simulink model "uncontrolled"  (R2021a)
settings: Solver=ode15s  StartTime=0  StopTime=6043.3926  MaxStep=0.0038168  RelTol=1e-8  AbsTol=1e-8
values from neighbouring files (symbols this model uses):
  I_x = 91.6*1e-2    (= 0.916)    [DATA.m]
  I_y = 25.1*1e-2    (= 0.251)    [DATA.m]
  I_z = 100.9*1e-2    (= 1.009)    [DATA.m]
  mag_ind = [0.1 0.5 0.1]'    [DATA.m]
  mu_E = 398600    [DATA.m]
  n_sun = 2*pi/365/24/3600    (= 1.99238499086e-07)    [DATA.m]
  phi0_312 = -atan(A_313_0(2,1)/A_313_0(2,2))    [DATA.m]
  phi0_313 = deg2rad(9.7)    [DATA.m]
  psi0_312 = -atan(A_313_0(1,3)/A_313_0(3,3))    [DATA.m]
  psi0_313 = deg2rad(6)    [DATA.m]
  R_E = 6.3710e3    (= 6371)    [DATA.m]
  th0_312 = asin(A_313_0(2,3))    [DATA.m]
  th0_313 = deg2rad(19)    [DATA.m]
  w_E = 2*pi/24/3600    (= 7.27220521664e-05)    [DATA.m]
undefined symbols (not defined in the file or in its folder): orbit, SRP
libraries: lib x11, vrlib x1, simulink_extras x1
settings Model: Creator=dvd33  LastModifiedBy=dvd33
settings SolverCC: AlgebraicLoopSolver=TrustRegion  ODENIntegrationMethod=ode4
settings DebuggingCC: IgnoredZcDiagnostic=none  SFMachineParentedDataDiag=warning

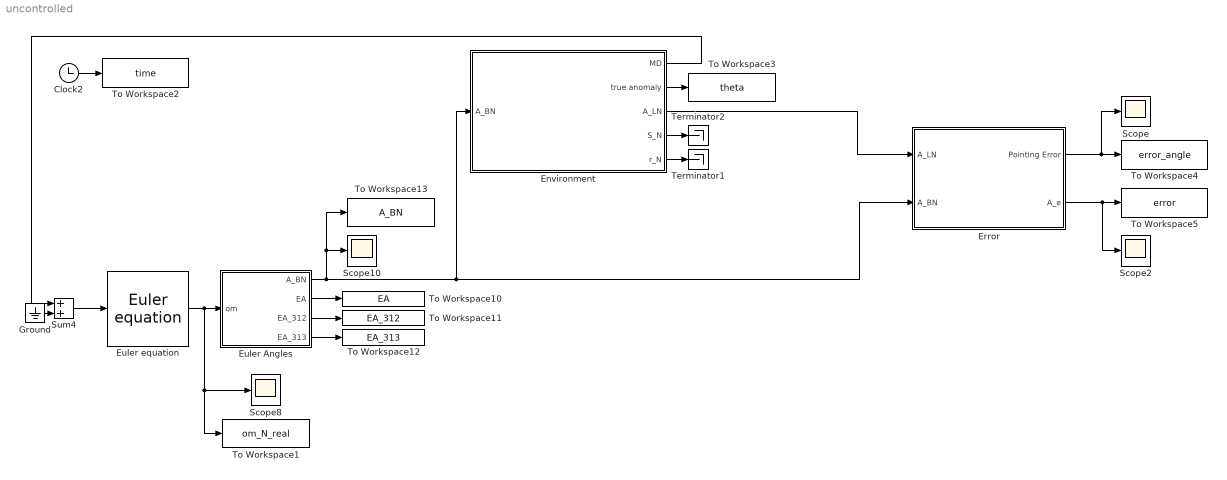
== system uncontrolled ==
  Clock2 : Clock
  Environment : Subsystem
  Error : Subsystem
  Euler Angles : Subsystem
  Euler equation : lib/Euler equation  SystemSampleTime=-1  VariantActivationTime=update diagram  Latency=0  AutoFrameSizeCalculation=off
  Ground : Ground
  Scope{,2,8,10} (4 alike) : Scope
  Sum4 : Sum
  Terminator1 : Terminator
  Terminator2 : Terminator
  To Workspace1 : ToWorkspace  VariableName=om_N_real  SampleTime=-1
  To Workspace10 : ToWorkspace  VariableName=EA  SampleTime=-1
  To Workspace11 : ToWorkspace  VariableName=EA_312  SampleTime=-1
  To Workspace12 : ToWorkspace  VariableName=EA_313  SampleTime=-1
  To Workspace13 : ToWorkspace  VariableName=A_BN  SampleTime=-1
  To Workspace2 : ToWorkspace  VariableName=time  SampleTime=-1
  To Workspace3 : ToWorkspace  VariableName=theta  SampleTime=-1
  To Workspace4 : ToWorkspace  VariableName=error_angle  SampleTime=-1
  To Workspace5 : ToWorkspace  VariableName=error  SampleTime=-1
  wires:
  Euler Angles/3(EA_312) -> To Workspace11/1
  Euler Angles/4(EA_313) -> To Workspace12/1
  Euler Angles/2(EA) -> To Workspace10/1
  Euler equation/1 -> Euler Angles/1(om), To Workspace1/1, Scope8/1
  Environment/2(true anomaly) -> To Workspace3/1
  Environment/3(A_LN) -> Error/1(A_LN)
  Environment/1(MD) -> Sum4/1
  Error/2(A_e) -> Scope2/1, To Workspace5/1
  Euler Angles/1(A_BN) -> Environment/1(A_BN), Error/2(A_BN), To Workspace13/1, Scope10/1
  Error/1(Pointing Error) -> To Workspace4/1, Scope/1
  Clock2/1 -> To Workspace2/1
  Sum4/1 -> Euler equation/1
  Ground/1 -> Sum4/2
  Environment/4(S_N) -> Terminator2/1
  Environment/5(r_N) -> Terminator1/1

== system uncontrolled/Environment ==
  A_BN : Inport
  A_BN1 : InportShadow
  Disturbance torques : Subsystem
  Orbit and Sun : Subsystem
  MD : Outport
  true anomaly : Outport  Port=2
  A_LN : Outport  Port=3
  S_N : Outport  Port=4
  r_N : Outport  Port=5
  wires:
  Orbit and Sun/1(r_N) -> r_N/1, Disturbance torques/1(r_N)
  Orbit and Sun/3(true anomaly) -> true anomaly/1
  A_BN/1 -> Orbit and Sun/1(A_BN)
  Disturbance torques/1(MD) -> MD/1
  Orbit and Sun/2(A_LN) -> A_LN/1, Disturbance torques/2(A_LN)
  Orbit and Sun/4(S_B) -> Disturbance torques/4(S_B)
  Orbit and Sun/5(S_N) -> S_N/1
  A_BN1/1 -> Disturbance torques/3(A_BN)

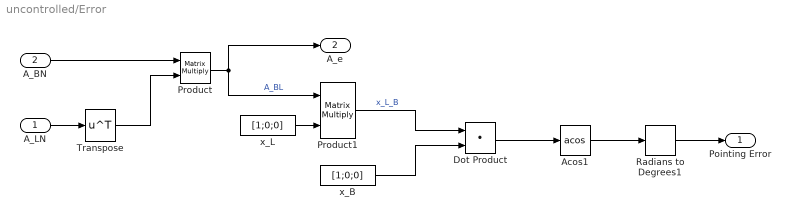
== system uncontrolled/Error ==
  A_LN : Inport
  A_BN : Inport  Port=2
  Acos1 : Trigonometry  Operator=acos
  Dot Product : DotProduct  InputSameDT=on  OutDataTypeStr=Inherit: Inherit via internal rule
  Product : Product  Multiplication=Matrix(*)
  Product1 : Product  Multiplication=Matrix(*)
  Radians to Degrees1 : simulink_extras/Transformations/Radians to Degrees
  Transpose : Math  Operator=transpose  SaturateOnIntegerOverflow=on
  x_B : Constant  Value=[1;0;0]
  x_L : Constant  Value=[1;0;0]
  Pointing Error : Outport
  A_e : Outport  Port=2
  wires:
  A_LN/1 -> Transpose/1
  A_BN/1 -> Product/1
  Transpose/1 -> Product/2
  Product/1 -> Product1/1, A_e/1  "A_BL"
  Radians to Degrees1/1 -> Pointing Error/1
  x_L/1 -> Product1/2
  Dot Product/1 -> Acos1/1
  Acos1/1 -> Radians to Degrees1/1
  Product1/1 -> Dot Product/1  "x_L_B"
  x_B/1 -> Dot Product/2

== system uncontrolled/Euler Angles ==
  om : Inport
  312 : Subsystem  TreatAsAtomicUnit=on
  313 : Subsystem  TreatAsAtomicUnit=on
  Abs : Abs
  SWITCH : Subsystem
  Selector2 : Selector  NumberOfDimensions=2  InputPortWidth=3,3  IndexOptions=Index vector (dialog),Index vector (dialog)  Indices=3,3  OutputSizes=1,1
  A_BN : Outport
  EA : Outport  Port=2
  EA_312 : Outport  Port=3
  EA_313 : Outport  Port=4
  wires:
  om/1 -> 313/1(om), 312/1(om)
  Selector2/1 -> Abs/1  "cos(th)"
  312/2(EA) -> SWITCH/2(EA_312), EA_312/1
  313/2(EA) -> SWITCH/5(EA_313), EA_313/1
  313/1(A_BN_313) -> Selector2/1, SWITCH/4(A_BN_313)
  312/1(A_BN_312) -> SWITCH/1(A_BN_312)
  Abs/1 -> SWITCH/3(u1)
  SWITCH/1(EA) -> EA/1
  SWITCH/2(A_BN) -> A_BN/1

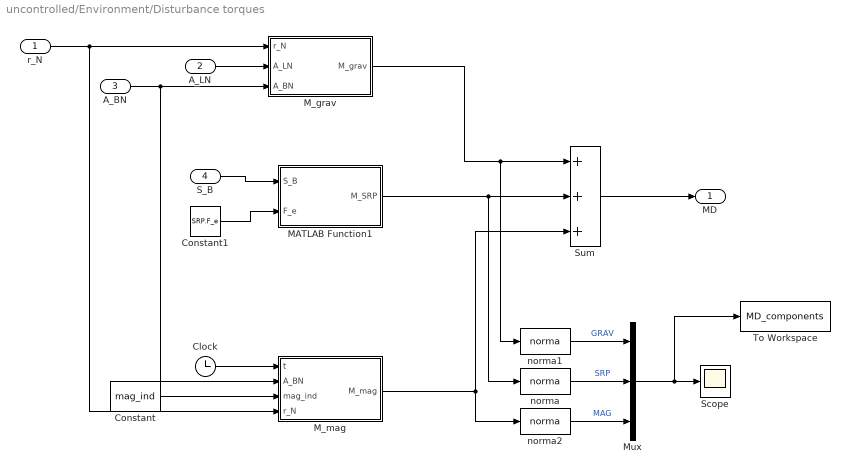
== system uncontrolled/Environment/Disturbance torques ==
  r_N : Inport
  A_LN : Inport  Port=2
  A_BN : Inport  Port=3
  S_B : Inport  Port=4
  Clock : Clock
  Constant : Constant  Value=mag_ind
  Constant1 : Constant  Value=SRP.F_e
  MATLAB Function1 : MATLAB Function  TreatAsAtomicUnit=on
  M_grav : Subsystem
  M_mag : Subsystem
  Mux : Mux  Inputs=3
  Scope : Scope
  Sum : Sum  Inputs=+++
  To Workspace : ToWorkspace  VariableName=MD_components  SampleTime=-1
  norma : lib/norma  SystemSampleTime=-1  VariantActivationTime=update diagram  Latency=0  AutoFrameSizeCalculation=off
  norma1 : lib/norma  SystemSampleTime=-1  VariantActivationTime=update diagram  Latency=0  AutoFrameSizeCalculation=off
  norma2 : lib/norma  SystemSampleTime=-1  VariantActivationTime=update diagram  Latency=0  AutoFrameSizeCalculation=off
  MD : Outport
  wires:
  r_N/1 -> M_grav/1(r_N), M_mag/4(r_N)
  A_LN/1 -> M_grav/2(A_LN)
  A_BN/1 -> M_mag/2(A_BN), M_grav/3(A_BN)
  Sum/1 -> MD/1
  M_grav/1(M_grav) -> norma1/1, Sum/1
  S_B/1 -> MATLAB Function1/1(S_B)
  MATLAB Function1/1(M_SRP) -> Sum/2, norma/1
  M_mag/1(M_mag) -> norma2/1, Sum/3
  Clock/1 -> M_mag/1(t)
  Constant/1 -> M_mag/3(mag_ind)
  Mux/1 -> To Workspace/1, Scope/1
  norma1/1 -> Mux/1  "GRAV"
  norma2/1 -> Mux/3  "MAG"
  norma/1 -> Mux/2  "SRP"
  Constant1/1 -> MATLAB Function1/2(F_e)

== system uncontrolled/Environment/Orbit and Sun ==
  A_BN : Inport
  Clock : Clock
  Orbit : Subsystem
  Product : Product  Multiplication=Matrix(*)
  Subsystem : Subsystem
  Sun direction : Subsystem
  r_N : Outport
  A_LN : Outport  Port=2
  true anomaly : Outport  Port=3
  S_B : Outport  Port=4
  S_N : Outport  Port=5
  wires:
  A_BN/1 -> Product/1
  Orbit/2(true anomaly) -> Subsystem/1(theta), true anomaly/1
  Orbit/1(r_N) -> r_N/1
  Clock/1 -> Sun direction/1(t)
  Sun direction/1(S_N) -> Product/2, S_N/1
  Product/1 -> S_B/1
  Subsystem/1(A_LN) -> A_LN/1

== system uncontrolled/Euler Angles/312 ==
  om : Inport
  A_312 : Subsystem
  Angles 312 : Subsystem
  A_BN_312 : Outport
  EA : Outport  Port=2
  wires:
  Angles 312/1(EA) -> A_312/1(EA), EA/1
  om/1 -> Angles 312/1(om)
  A_312/1(A_BN_312) -> A_BN_312/1

== system uncontrolled/Euler Angles/313 ==
  om : Inport
  A_313 : Subsystem
  Angles 313 : Subsystem
  A_BN_313 : Outport
  EA : Outport  Port=2
  wires:
  Angles 313/1(EA) -> A_313/1(EA), EA/1
  A_313/1(A_BN_313) -> A_BN_313/1
  om/1 -> Angles 313/1(om)

== system uncontrolled/Euler Angles/SWITCH ==
  A_BN_312 : Inport
  EA_312 : Inport  Port=2
  u1 : Inport  Port=3
  A_BN_313 : Inport  Port=4
  EA_313 : Inport  Port=5
  Switch : Switch  Criteria=u2 > Threshold  Threshold=0.9999
  Switch2 : Switch  Criteria=u2 > Threshold  Threshold=0.9999
  u1_1 : InportShadow  Port=3
  EA : Outport
  A_BN : Outport  Port=2
  wires:
  u1/1 -> Switch2/2
  Switch2/1 -> A_BN/1
  Switch/1 -> EA/1
  EA_312/1 -> Switch/1
  EA_313/1 -> Switch/3
  A_BN_312/1 -> Switch2/1
  A_BN_313/1 -> Switch2/3
  u1_1/1 -> Switch/2

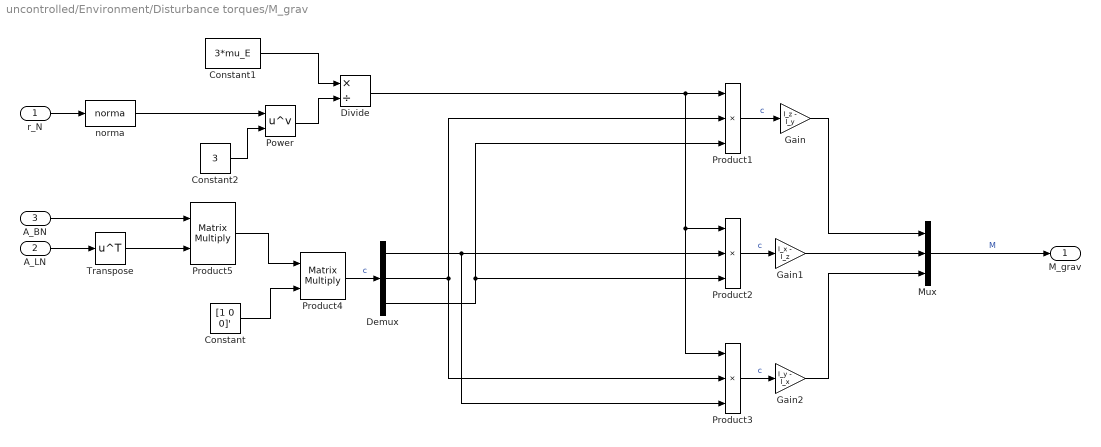
== system uncontrolled/Environment/Disturbance torques/M_grav ==
  r_N : Inport
  A_LN : Inport  Port=2
  A_BN : Inport  Port=3
  Constant : Constant  Value=[1 0 0]'
  Constant1 : Constant  Value=3*mu_E
  Constant2 : Constant  Value=3
  Demux : Demux  Outputs=3
  Divide : Product  Inputs=*/
  Gain : Gain  Gain=I_z - I_y
  Gain1 : Gain  Gain=I_x - I_z
  Gain2 : Gain  Gain=I_y - I_x
  Mux : Mux  Inputs=3
  Power : Math  Operator=pow  SaturateOnIntegerOverflow=on
  Product1 : Product  Inputs=3
  Product2 : Product  Inputs=3
  Product3 : Product  Inputs=3
  Product4 : Product  Multiplication=Matrix(*)
  Product5 : Product  Multiplication=Matrix(*)
  Transpose : Math  Operator=transpose  SaturateOnIntegerOverflow=on
  norma : lib/norma  SystemSampleTime=-1  VariantActivationTime=update diagram  Latency=0  AutoFrameSizeCalculation=off
  M_grav : Outport
  wires:
  A_LN/1 -> Transpose/1
  Demux/1 -> Product2/2, Product3/3
  Product2/1 -> Gain1/1  "c"
  Constant/1 -> Product4/2
  Product5/1 -> Product4/1
  Transpose/1 -> Product5/2
  Mux/1 -> M_grav/1  "M"
  Product1/1 -> Gain/1  "c"
  Constant1/1 -> Divide/1
  Product3/1 -> Gain2/1  "c"
  Power/1 -> Divide/2
  Demux/2 -> Product3/2, Product1/2
  Divide/1 -> Product1/1, Product2/1, Product3/1
  Constant2/1 -> Power/2
  Demux/3 -> Product1/3, Product2/3
  Product4/1 -> Demux/1  "c"
  A_BN/1 -> Product5/1
  r_N/1 -> norma/1
  norma/1 -> Power/1
  Gain/1 -> Mux/1
  Gain1/1 -> Mux/2
  Gain2/1 -> Mux/3

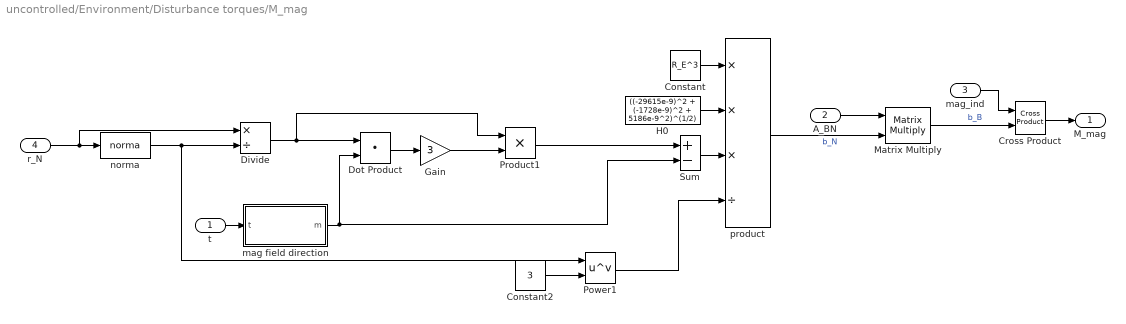
== system uncontrolled/Environment/Disturbance torques/M_mag ==
  t : Inport
  A_BN : Inport  Port=2
  mag_ind : Inport  Port=3
  r_N : Inport  Port=4
  Constant : Constant  Value=R_E^3
  Constant2 : Constant  Value=3
  Cross Product : vrlib/Utilities/Cross Product
  Divide : Product  Inputs=*/
  Dot Product : DotProduct  InputSameDT=on  OutDataTypeStr=Inherit: Inherit via internal rule
  Gain : Gain  Gain=3
  H0 : Constant  Value=((-29615e-9)^2 + (-1728e-9)^2 + 5186e-9^2)^(1/2)
  Matrix Multiply : Product  Multiplication=Matrix(*)
  Power1 : Math  Operator=pow  SaturateOnIntegerOverflow=on
  Product1 : Product
  Sum : Sum  Inputs=+-
  mag field direction : Subsystem
  norma : lib/norma  SystemSampleTime=-1  VariantActivationTime=update diagram  Latency=0  AutoFrameSizeCalculation=off
  product : Product  Inputs=***/
  M_mag : Outport
  wires:
  t/1 -> mag field direction/1(t)
  A_BN/1 -> Matrix Multiply/1
  Constant/1 -> product/1
  Power1/1 -> product/4
  Constant2/1 -> Power1/2
  norma/1 -> Power1/1, Divide/2
  Divide/1 -> Product1/1, Dot Product/1
  H0/1 -> product/2
  Dot Product/1 -> Gain/1
  Gain/1 -> Product1/2
  Sum/1 -> product/3
  product/1 -> Matrix Multiply/2  "b_N"
  r_N/1 -> Divide/1, norma/1
  mag field direction/1(m) -> Dot Product/2, Sum/2
  Cross Product/1 -> M_mag/1
  Product1/1 -> Sum/1
  Matrix Multiply/1 -> Cross Product/2  "b_B"
  mag_ind/1 -> Cross Product/1

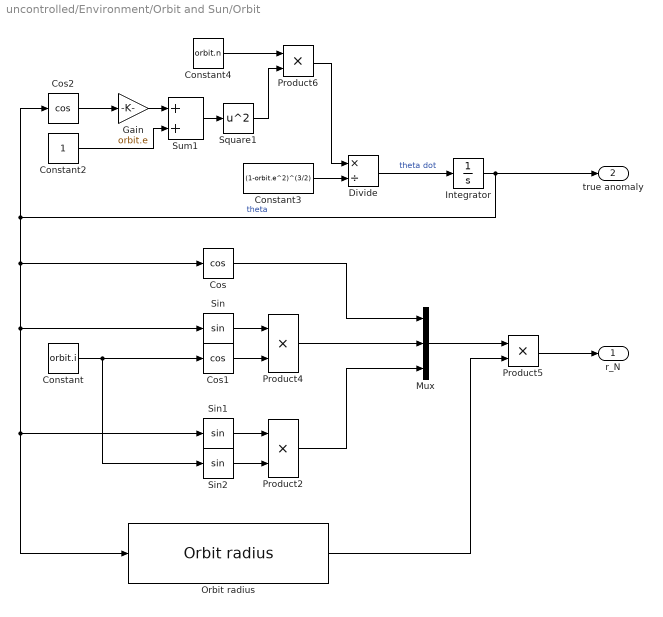
== system uncontrolled/Environment/Orbit and Sun/Orbit ==
  Constant : Constant  Value=orbit.i
  Constant2 : Constant
  Constant3 : Constant  Value=(1-orbit.e^2)^(3/2)
  Constant4 : Constant  Value=orbit.n
  Cos : Trigonometry  Operator=cos
  Cos1 : Trigonometry  Operator=cos
  Cos2 : Trigonometry  Operator=cos
  Divide : Product  Inputs=*/
  Gain : Gain  Gain=orbit.e
  Integrator : Integrator  InitialCondition=orbit.theta0
  Mux : Mux  Inputs=3
  Orbit radius : lib/Orbit radius  SystemSampleTime=-1  VariantActivationTime=update diagram  Latency=0  AutoFrameSizeCalculation=off
      link override Constant: Value=orbit.a*(1-orbit.e^2)
      link override eccentricity: Value=orbit.e
  Product{2,4..6} (4 alike) : Product
  Sin : Trigonometry
  Sin1 : Trigonometry
  Sin2 : Trigonometry
  Square1 : Math  Operator=square  SaturateOnIntegerOverflow=on
  Sum1 : Sum
  r_N : Outport
  true anomaly : Outport  Port=2
  wires:
  Divide/1 -> Integrator/1  "theta dot"
  Integrator/1 -> true anomaly/1, Cos2/1, Sin/1, Orbit radius/1, Sin1/1, Cos/1  "theta"
  Product2/1 -> Mux/3
  Constant2/1 -> Sum1/2
  Product5/1 -> r_N/1
  Sin1/1 -> Product2/1
  Orbit radius/1 -> Product5/2
  Constant4/1 -> Product6/1
  Square1/1 -> Product6/2
  Sum1/1 -> Square1/1
  Gain/1 -> Sum1/1
  Cos1/1 -> Product4/2
  Product4/1 -> Mux/2
  Cos2/1 -> Gain/1
  Product6/1 -> Divide/1
  Constant3/1 -> Divide/2
  Constant/1 -> Sin2/1, Cos1/1
  Sin2/1 -> Product2/2
  Cos/1 -> Mux/1
  Mux/1 -> Product5/1
  Sin/1 -> Product4/1

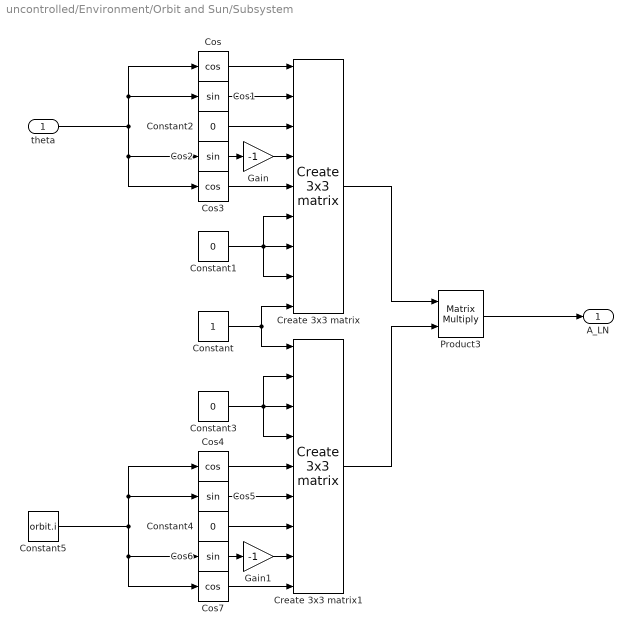
== system uncontrolled/Environment/Orbit and Sun/Subsystem ==
  theta : Inport
  Constant : Constant
  Constant{1..4} (4 alike) : Constant  Value=0
  Constant5 : Constant  Value=orbit.i
  Cos{,3..4,7} (4 alike) : Trigonometry  Operator=cos
  Cos{1..2,5..6} (4 alike) : Trigonometry
  Create 3x3 matrix : lib/Create 3x3 matrix  SystemSampleTime=-1  VariantActivationTime=update diagram  Latency=0  AutoFrameSizeCalculation=off
  Create 3x3 matrix1 : lib/Create 3x3 matrix  SystemSampleTime=-1  VariantActivationTime=update diagram  Latency=0  AutoFrameSizeCalculation=off
  Gain : Gain  Gain=-1
  Gain1 : Gain  Gain=-1
  Product3 : Product  Multiplication=Matrix(*)
  A_LN : Outport
  wires:
  Create 3x3 matrix1/1 -> Product3/2
  Create 3x3 matrix/1 -> Product3/1
  Product3/1 -> A_LN/1
  Cos/1 -> Create 3x3 matrix/1
  Cos1/1 -> Create 3x3 matrix/2
  Cos3/1 -> Create 3x3 matrix/5
  Cos2/1 -> Gain/1
  Gain/1 -> Create 3x3 matrix/4
  Constant/1 -> Create 3x3 matrix1/1, Create 3x3 matrix/9
  Constant1/1 -> Create 3x3 matrix/6, Create 3x3 matrix/7, Create 3x3 matrix/8
  Constant2/1 -> Create 3x3 matrix/3
  Constant3/1 -> Create 3x3 matrix1/2, Create 3x3 matrix1/3, Create 3x3 matrix1/4
  Cos5/1 -> Create 3x3 matrix1/6
  Cos4/1 -> Create 3x3 matrix1/5
  Constant4/1 -> Create 3x3 matrix1/7
  Cos7/1 -> Create 3x3 matrix1/9
  Cos6/1 -> Gain1/1
  Gain1/1 -> Create 3x3 matrix1/8
  theta/1 -> Cos2/1, Cos3/1, Cos/1, Cos1/1
  Constant5/1 -> Cos6/1, Cos7/1, Cos5/1, Cos4/1

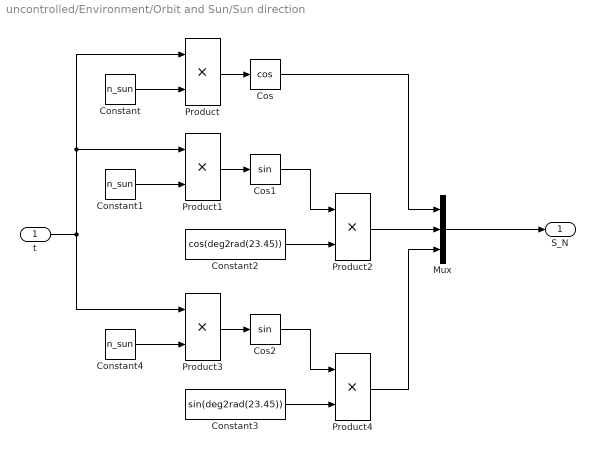
== system uncontrolled/Environment/Orbit and Sun/Sun direction ==
  t : Inport
  Constant : Constant  Value=n_sun
  Constant1 : Constant  Value=n_sun
  Constant2 : Constant  Value=cos(deg2rad(23.45))
  Constant3 : Constant  Value=sin(deg2rad(23.45))
  Constant4 : Constant  Value=n_sun
  Cos : Trigonometry  Operator=cos
  Cos1 : Trigonometry
  Cos2 : Trigonometry
  Mux : Mux  Inputs=3
  Product{,1..4} (5 alike) : Product
  S_N : Outport
  wires:
  Mux/1 -> S_N/1
  Constant/1 -> Product/2
  Product/1 -> Cos/1
  Cos/1 -> Mux/1
  Product1/1 -> Cos1/1
  Constant1/1 -> Product1/2
  Cos1/1 -> Product2/1
  Constant2/1 -> Product2/2
  Product2/1 -> Mux/2
  t/1 -> Product3/1, Product1/1, Product/1
  Product4/1 -> Mux/3
  Cos2/1 -> Product4/1
  Constant4/1 -> Product3/2
  Product3/1 -> Cos2/1
  Constant3/1 -> Product4/2

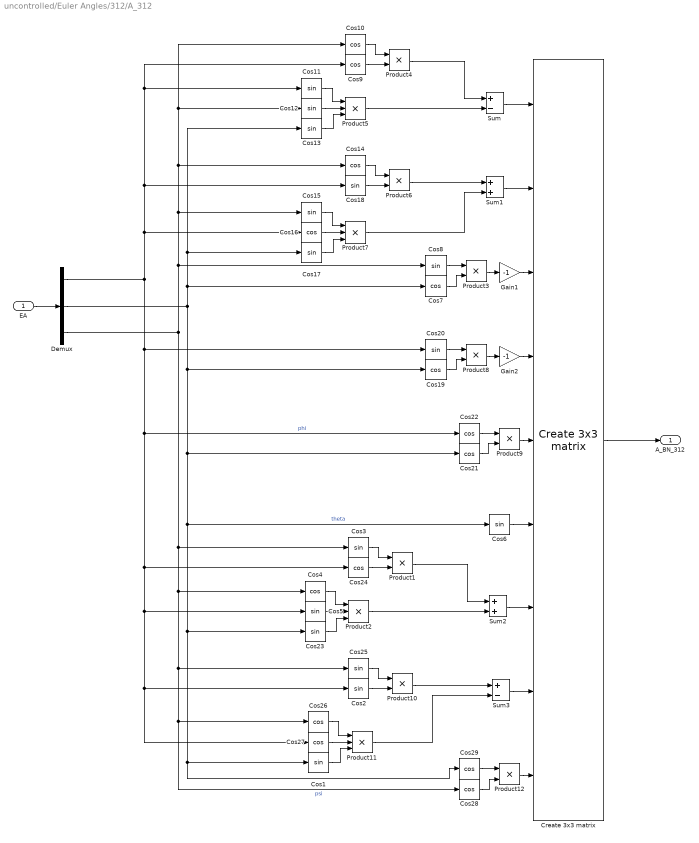
== system uncontrolled/Euler Angles/312/A_312 ==
  EA : Inport
  Cos{1..3,5..6,8,11..13,15,17..18,20,23,25} (15 alike) : Trigonometry
  Cos{4,7,9..10,14,16,19,21..22,24,26..29} (14 alike) : Trigonometry  Operator=cos
  Create 3x3 matrix : lib/Create 3x3 matrix  SystemSampleTime=-1  VariantActivationTime=update diagram  Latency=0  AutoFrameSizeCalculation=off
  Demux : Demux  Outputs=3
  Gain1 : Gain  Gain=-1
  Gain2 : Gain  Gain=-1
  Product{1,3..4,6,8..10,12} (8 alike) : Product
  Product{2,5,7,11} (4 alike) : Product  Inputs=3
  Sum : Sum  Inputs=+-
  Sum1 : Sum
  Sum2 : Sum
  Sum3 : Sum  Inputs=+-
  A_BN_312 : Outport
  wires:
  EA/1 -> Demux/1
  Demux/1 -> Cos24/1, Cos5/1, Cos27/1, Cos2/1, Cos22/1, Cos20/1, Cos16/1, Cos18/1, Cos9/1, Cos11/1  "phi"
  Demux/3 -> Cos8/1, Cos15/1, Cos14/1, Cos10/1, Cos12/1, Cos3/1, Cos4/1, Cos25/1, Cos26/1, Cos28/1  "psi"
  Demux/2 -> Cos1/1, Cos29/1, Cos23/1, Cos6/1, Cos21/1, Cos19/1, Cos7/1, Cos13/1, Cos17/1  "theta"
  Product12/1 -> Create 3x3 matrix/9
  Cos29/1 -> Product12/1
  Cos28/1 -> Product12/2
  Sum3/1 -> Create 3x3 matrix/8
  Cos27/1 -> Product11/2
  Product11/1 -> Sum3/2
  Cos25/1 -> Product10/1
  Product10/1 -> Sum3/1
  Cos2/1 -> Product10/2
  Cos26/1 -> Product11/1
  Cos1/1 -> Product11/3
  Cos23/1 -> Product2/3
  Cos4/1 -> Product2/1
  Product2/1 -> Sum2/2
  Cos5/1 -> Product2/2
  Cos24/1 -> Product1/2
  Product1/1 -> Sum2/1
  Cos3/1 -> Product1/1
  Sum2/1 -> Create 3x3 matrix/7
  Product9/1 -> Create 3x3 matrix/5
  Cos22/1 -> Product9/1
  Cos21/1 -> Product9/2
  Product8/1 -> Gain2/1
  Cos20/1 -> Product8/1
  Cos19/1 -> Product8/2
  Gain1/1 -> Create 3x3 matrix/3
  Create 3x3 matrix/1 -> A_BN_312/1
  Product6/1 -> Sum1/1
  Sum/1 -> Create 3x3 matrix/1
  Cos7/1 -> Product3/2
  Cos8/1 -> Product3/1
  Gain2/1 -> Create 3x3 matrix/4
  Cos9/1 -> Product4/2
  Sum1/1 -> Create 3x3 matrix/2
  Product4/1 -> Sum/1
  Cos12/1 -> Product5/2
  Product5/1 -> Sum/2
  Cos11/1 -> Product5/1
  Cos17/1 -> Product7/3
  Cos14/1 -> Product6/1
  Cos6/1 -> Create 3x3 matrix/6
  Cos13/1 -> Product5/3
  Product7/1 -> Sum1/2
  Product3/1 -> Gain1/1
  Cos16/1 -> Product7/2
  Cos15/1 -> Product7/1
  Cos18/1 -> Product6/2
  Cos10/1 -> Product4/1

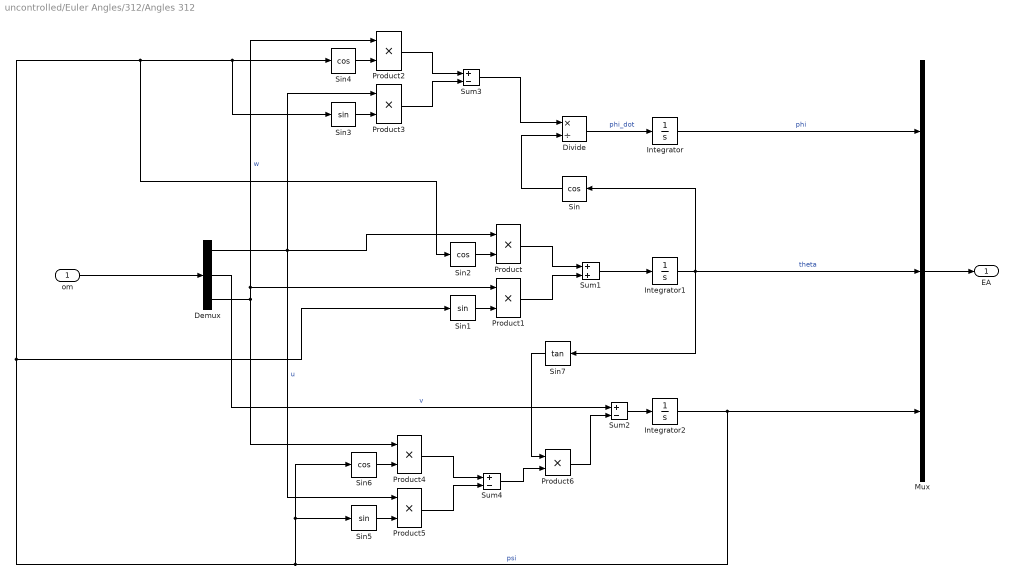
== system uncontrolled/Euler Angles/312/Angles 312 ==
  om : Inport
  Demux : Demux  Outputs=3
  Divide : Product  Inputs=*/
  Integrator : Integrator  InitialCondition=phi0_312  WrapState=on
  Integrator1 : Integrator  InitialCondition=th0_312  WrapState=on
  Integrator2 : Integrator  InitialCondition=psi0_312  WrapState=on
  Mux : Mux  Inputs=3
  Product{,1..6} (7 alike) : Product
  Sin{,2,4,6} (4 alike) : Trigonometry  Operator=cos
  Sin1 : Trigonometry
  Sin3 : Trigonometry
  Sin5 : Trigonometry
  Sin7 : Trigonometry  Operator=tan
  Sum1 : Sum
  Sum2 : Sum  Inputs=+-
  Sum3 : Sum  Inputs=+-
  Sum4 : Sum  Inputs=+-
  EA : Outport
  wires:
  Mux/1 -> EA/1
  Sum4/1 -> Product6/2
  Demux/2 -> Sum2/1  "v"
  Integrator2/1 -> Mux/3, Sin6/1, Sin5/1, Sin3/1, Sin4/1, Sin2/1, Sin1/1  "psi"
  Demux/3 -> Product2/1, Product1/1, Product4/1  "w"
  Sin4/1 -> Product2/2
  Product1/1 -> Sum1/2
  Sin1/1 -> Product1/2
  Sin3/1 -> Product3/2
  Divide/1 -> Integrator/1  "phi_dot"
  Sum1/1 -> Integrator1/1
  Product6/1 -> Sum2/2
  Sin5/1 -> Product5/2
  om/1 -> Demux/1
  Product4/1 -> Sum4/1
  Sum3/1 -> Divide/1
  Product5/1 -> Sum4/2
  Sin6/1 -> Product4/2
  Integrator1/1 -> Sin/1, Mux/2, Sin7/1  "theta"
  Integrator/1 -> Mux/1  "phi"
  Product3/1 -> Sum3/2
  Demux/1 -> Product3/1, Product/1, Product5/1  "u"
  Sin/1 -> Divide/2
  Product/1 -> Sum1/1
  Sin7/1 -> Product6/1
  Product2/1 -> Sum3/1
  Sum2/1 -> Integrator2/1
  Sin2/1 -> Product/2

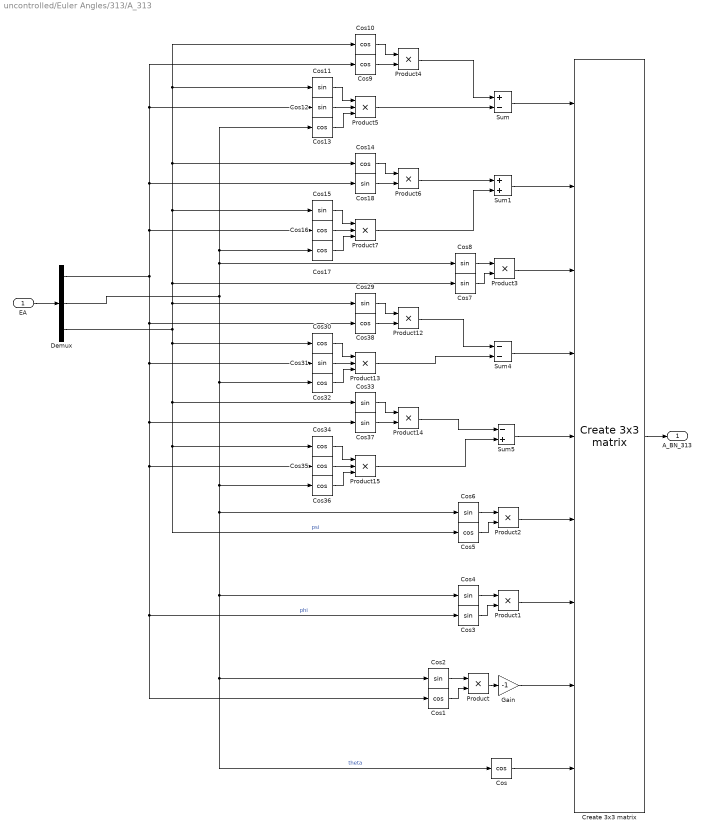
== system uncontrolled/Euler Angles/313/A_313 ==
  EA : Inport
  Cos{,1,5,9..10,13..14,16..17,30,32,34..36,38} (15 alike) : Trigonometry  Operator=cos
  Cos{2..4,6..8,11..12,15,18,29,31,33,37} (14 alike) : Trigonometry
  Create 3x3 matrix : lib/Create 3x3 matrix  SystemSampleTime=-1  VariantActivationTime=update diagram  Latency=0  AutoFrameSizeCalculation=off
  Demux : Demux  Outputs=3
  Gain : Gain  Gain=-1
  Product{,1..4,6,12,14} (8 alike) : Product
  Product{5,7,13,15} (4 alike) : Product  Inputs=3
  Sum : Sum  Inputs=+-
  Sum1 : Sum
  Sum4 : Sum  Inputs=--
  Sum5 : Sum  Inputs=-+
  A_BN_313 : Outport
  wires:
  EA/1 -> Demux/1
  Cos10/1 -> Product4/1
  Demux/2 -> Cos32/1, Cos6/1, Cos4/1, Cos/1, Cos2/1, Cos36/1, Cos8/1, Cos17/1, Cos13/1  "theta"
  Product15/1 -> Sum5/2
  Cos18/1 -> Product6/2
  Demux/1 -> Cos38/1, Cos37/1, Cos3/1, Cos1/1, Cos35/1, Cos31/1, Cos9/1, Cos12/1, Cos18/1, Cos16/1  "phi"
  Cos15/1 -> Product7/1
  Cos36/1 -> Product15/3
  Cos16/1 -> Product7/2
  Cos5/1 -> Product2/2
  Demux/3 -> Cos29/1, Cos7/1, Cos15/1, Cos14/1, Cos10/1, Cos11/1, Cos30/1, Cos5/1, Cos34/1, Cos33/1  "psi"
  Cos38/1 -> Product12/2
  Product3/1 -> Create 3x3 matrix/3
  Product7/1 -> Sum1/2
  Cos13/1 -> Product5/3
  Cos4/1 -> Product1/1
  Cos6/1 -> Product2/1
  Cos14/1 -> Product6/1
  Product2/1 -> Create 3x3 matrix/6
  Product14/1 -> Sum5/1
  Cos37/1 -> Product14/2
  Product/1 -> Gain/1
  Cos17/1 -> Product7/3
  Cos29/1 -> Product12/1
  Cos11/1 -> Product5/1
  Cos33/1 -> Product14/1
  Product12/1 -> Sum4/1
  Product5/1 -> Sum/2
  Cos12/1 -> Product5/2
  Cos2/1 -> Product/1
  Product4/1 -> Sum/1
  Cos3/1 -> Product1/2
  Sum1/1 -> Create 3x3 matrix/2
  Cos9/1 -> Product4/2
  Sum5/1 -> Create 3x3 matrix/5
  Gain/1 -> Create 3x3 matrix/8
  Sum4/1 -> Create 3x3 matrix/4
  Cos8/1 -> Product3/1
  Cos32/1 -> Product13/3
  Cos7/1 -> Product3/2
  Sum/1 -> Create 3x3 matrix/1
  Product13/1 -> Sum4/2
  Cos34/1 -> Product15/1
  Cos31/1 -> Product13/2
  Cos/1 -> Create 3x3 matrix/9
  Product6/1 -> Sum1/1
  Create 3x3 matrix/1 -> A_BN_313/1
  Product1/1 -> Create 3x3 matrix/7
  Cos35/1 -> Product15/2
  Cos30/1 -> Product13/1
  Cos1/1 -> Product/2

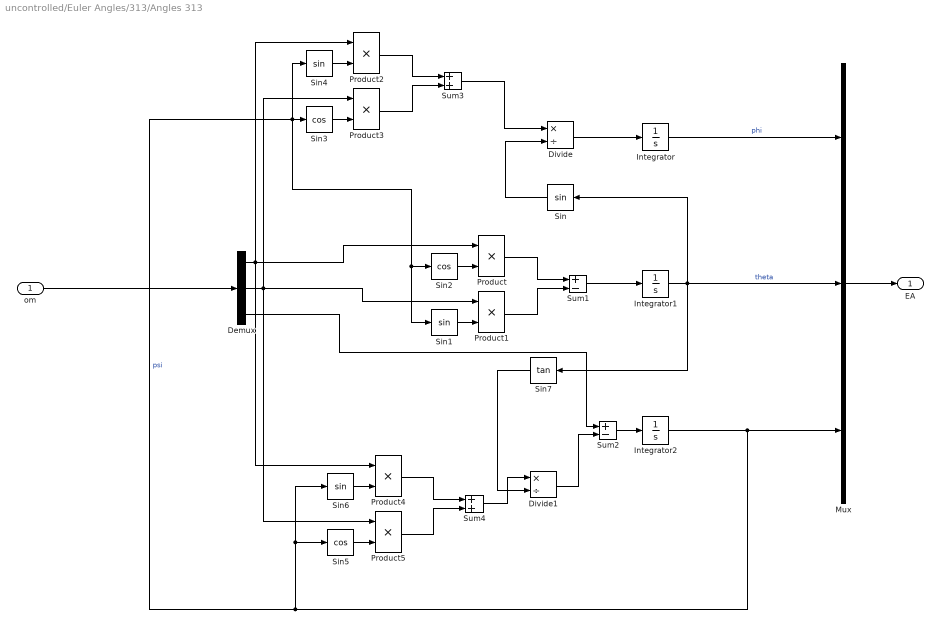
== system uncontrolled/Euler Angles/313/Angles 313 ==
  om : Inport
  Demux : Demux  Outputs=3
  Divide : Product  Inputs=*/
  Divide1 : Product  Inputs=*/
  Integrator : Integrator  InitialCondition=phi0_313  WrapState=on
  Integrator1 : Integrator  InitialCondition=th0_313  WrapState=on
  Integrator2 : Integrator  InitialCondition=psi0_313  WrapState=on
  Mux : Mux  Inputs=3
  Product{,1..5} (6 alike) : Product
  Sin{,1,4,6} (4 alike) : Trigonometry
  Sin2 : Trigonometry  Operator=cos
  Sin3 : Trigonometry  Operator=cos
  Sin5 : Trigonometry  Operator=cos
  Sin7 : Trigonometry  Operator=tan
  Sum1 : Sum  Inputs=+-
  Sum2 : Sum  Inputs=+-
  Sum3 : Sum
  Sum4 : Sum
  EA : Outport
  wires:
  Integrator1/1 -> Sin/1, Mux/2, Sin7/1  "theta"
  Mux/1 -> EA/1
  Sin2/1 -> Product/2
  Sum2/1 -> Integrator2/1
  Product2/1 -> Sum3/1
  Sin7/1 -> Divide1/2
  Product/1 -> Sum1/1
  Sin/1 -> Divide/2
  Demux/1 -> Product/1, Product2/1, Product4/1
  Product3/1 -> Sum3/2
  Integrator/1 -> Mux/1  "phi"
  Sin6/1 -> Product4/2
  Product5/1 -> Sum4/2
  Sum3/1 -> Divide/1
  Product4/1 -> Sum4/1
  om/1 -> Demux/1
  Sum4/1 -> Divide1/1
  Sin5/1 -> Product5/2
  Divide1/1 -> Sum2/2
  Sum1/1 -> Integrator1/1
  Divide/1 -> Integrator/1
  Demux/2 -> Product3/1, Product5/1, Product1/1
  Sin3/1 -> Product3/2
  Sin1/1 -> Product1/2
  Product1/1 -> Sum1/2
  Sin4/1 -> Product2/2
  Demux/3 -> Sum2/1
  Integrator2/1 -> Mux/3, Sin2/1, Sin1/1, Sin4/1, Sin3/1, Sin6/1, Sin5/1  "psi"

== system uncontrolled/Environment/Disturbance torques/M_mag/mag field direction ==
  t : Inport
  Constant : Constant  Value=cos(deg2rad(11.5))
  Constant1 : Constant  Value=sin(deg2rad(11.5))
  Constant2 : Constant  Value=w_E
  Cos : Trigonometry  Operator=cos
  Mux : Mux  Inputs=3
  Product : Product
  Product1 : Product
  Product2 : Product
  Sin : Trigonometry
  m : Outport
  wires:
  Constant/1 -> Mux/3
  Constant1/1 -> Product1/1, Product/1
  Product/1 -> Mux/1
  Product1/1 -> Mux/2
  Constant2/1 -> Product2/2
  t/1 -> Product2/1
  Cos/1 -> Product/2
  Sin/1 -> Product1/2
  Product2/1 -> Cos/1, Sin/1
  Mux/1 -> m/1

== matlab function uncontrolled/Environment/Disturbance torques/MATLAB Function1 ==
  data: S_B input; M_SRP output; F_e input
function M_SRP = fcn(S_B, F_e)
c = 3e8;
P = F_e/c;
M_SRP = [0; 0; 0];

N_B = [1 0 0; ...
       0 1 0; ...
       0 0 1; ...
      -1 0 0; ...
      0 -1 0; ...
      0 0 -1; ...
      0 1 0 ; ...
      0 1 0 ; ...
      0 -1 0; ...
      0 -1 0];
A = [4 6 6 4 6 6 10 10 10 10] * 0.1^2;  
b = [1 0 0; ...
     0 1 0; ...
     0 0 1.5; ...
    -1 0 0; ...
    0 -1 0; ...
    0 0 -1.5; ...
    2 0 0; ...
    2 0 0; ...
    2 0 0; ...
    2 0 0]*0.1;
b_CG = [1.8; 0; 0]*1e-2;
rho_s = [0.5 0.8]';
rho_d = [0.1 0.1]';


for i = 1:10
    N_Bi = N_B(i,:)';
    DOT = dot(S_B,N_Bi);
    if DOT>0
        j = 1;
        if i>6
            j = 2;
        end
        F = -P*A(i)*DOT*((1-rho_s(j))*S_B + (2*rho_s(j)*DOT+2/3*rho_d(j))*N_Bi);
        r = b(i,:)'- b_CG;
        M_SRP = M_SRP + cross(r,F); 
    end
end
